simulink model "stanley_ctrl"  (R2019a)
settings: Solver=FixedStepDiscrete  StartTime=0.0  StopTime=50.0  FixedStep=.1  RelTol=1e-3
libraries: drivingvehiclecontroller x1
settings Model: Creator=Cameron  LastModifiedBy=Cameron

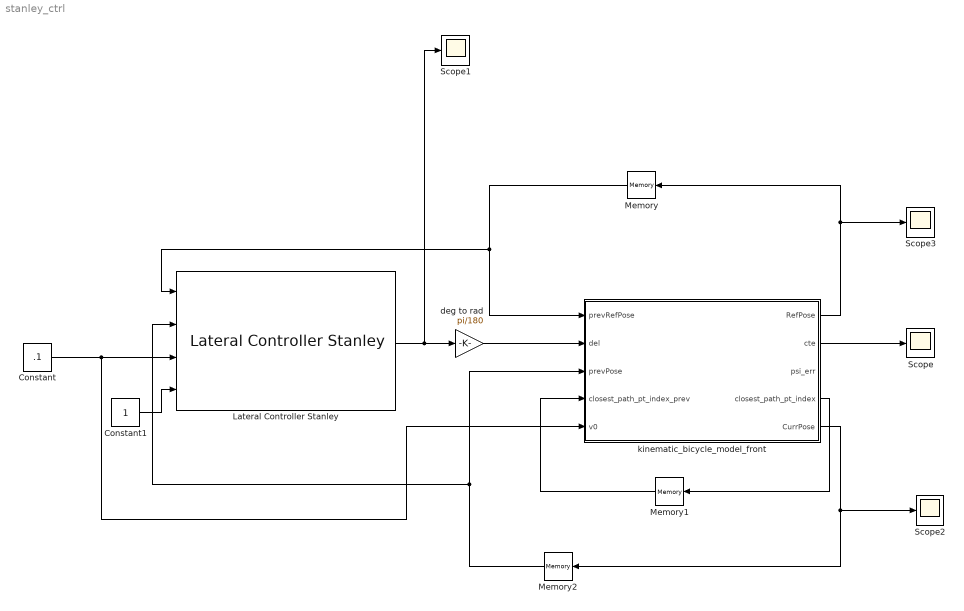
== system stanley_ctrl ==
  Constant : Constant  Value=.1
  Constant1 : Constant
  Lateral Controller Stanley : drivingvehiclecontroller/Lateral Controller Stanley  ModelType=Kinematic bicycle model  PositionGainF=5  PositionGainR=2.5  YawRateGain=0.2  DelayGain=0.2  VehicleMass=1575  Lf=1.2  Lr=1.6  TireStiffness=19000  Wheelbase=.46  MaxSteeringAngle=35
      settings: SourceProductName=Automated Driving Toolbox  SourceProductBaseCode=DR
  Memory : Memory  InitialCondition=[0 0 0]
  Memory1 : Memory  InitialCondition=1
  Memory2 : Memory  InitialCondition=[-.1 -.1 0]
  Scope{,1..3} (4 alike) : Scope
  deg to rad : Gain  Gain=pi/180
  kinematic_bicycle_model_front : MATLAB Function  TreatAsAtomicUnit=on
  wires:
  Lateral Controller Stanley/1 -> deg to rad/1, Scope1/1
  kinematic_bicycle_model_front/5(CurrPose) -> Scope2/1, Memory2/1
  kinematic_bicycle_model_front/1(RefPose) -> Scope3/1, Memory/1
  kinematic_bicycle_model_front/4(closest_path_pt_index) -> Memory1/1
  Memory1/1 -> kinematic_bicycle_model_front/4(closest_path_pt_index_prev)
  Constant/1 -> kinematic_bicycle_model_front/5(v0), Lateral Controller Stanley/3
  Constant1/1 -> Lateral Controller Stanley/4
  Memory/1 -> kinematic_bicycle_model_front/1(prevRefPose), Lateral Controller Stanley/1
  Memory2/1 -> kinematic_bicycle_model_front/3(prevPose), Lateral Controller Stanley/2
  kinematic_bicycle_model_front/2(cte) -> Scope/1
  deg to rad/1 -> kinematic_bicycle_model_front/2(del)

== matlab function stanley_ctrl/kinematic_bicycle_model_front ==
  data: prevRefPose input; RefPose output; cte output; psi_err output; closest_path_pt_index output; del input; CurrPose output; prevPose input; closest_path_pt_index_prev input; v0 input
function [RefPose, cte, psi_err, closest_path_pt_index, CurrPose] = fcn(prevRefPose, del, prevPose, closest_path_pt_index_prev, v0)

h = .1;  %sampling time
L = .46; %length of vehicle (m)

x = prevPose(1) + v0*cos(prevPose(3) + del)*h;
y = prevPose(2) + v0*sin(prevPose(3) + del)*h;
psi = prevPose(3) + (v0/L)*sin(del)*h;

CurrPose = zeros(1,3);

CurrPose(1) = x;
CurrPose(2) = y;
CurrPose(2) = psi;

% heading error and cross track error
heading_err = @(desired_psi, psi) desired_psi - psi;
crosstrack_err = @(path_y, y, path_x, x) sqrt((path_x-x)^2 + (path_y-y)^2);

% coords for entire path (we are given this by motion planner)
path_x = [.01:.01:10];
path_y = -sqrt(10^2 - path_x.^2) + 10;
path_heading = atan(path_x./sqrt(100-path_x.^2)); % heading of the path at every point (the atan of the path's derivative at every point)

RefPose = zeros(1,3);

i = 1;
while crosstrack_err(prevRefPose(2), y, prevRefPose(2), x) > crosstrack_err(path_y(closest_path_pt_index_prev+i), y, path_x(closest_path_pt_index_prev+i), x) 
    RefPose(1) = path_x(closest_path_pt_index_prev+i);
    RefPose(2) = path_y(closest_path_pt_index_prev+i);
    RefPose(3) = path_heading(closest_path_pt_index_prev+i);
    i = i+1;
end
closest_path_pt_index = closest_path_pt_index_prev + i; 
RefPose(3) = RefPose(3)*180/pi; %radians to degrees


psi_err = heading_err(path_heading(closest_path_pt_index), psi);
cte = crosstrack_err(path_y(closest_path_pt_index), y, path_x(closest_path_pt_index), x);
